simulink model "sgMdl_IO424_SynchroMeasurementTest"  (R2024b)
settings: Solver=FixedStepAuto  StartTime=0.0  StopTime=inf  RelTol=1e-3
libraries: dspsrcs4 x4, speedgoatlib_IO424 x2, speedgoatlib_IO107 x1
Description:
  | IO424 - Synchro Measurement
settings Model: ModifiedByFormat=Speedgoat  Creator=Speedgoat  LastModifiedBy=Speedgoat
settings SolverCC: ConcurrentTasks=on  PositivePriorityOrder=on
settings OptimizationCC: BlockReduction=off  OptimizeBlockIOStorage=off
settings DebuggingCC: TasksWithSamePriorityMsg=none
settings HardwareCC: ProdBitPerLong=64  ProdLongLongMode=on  ProdHWDeviceType=Intel->x86-64 (Linux 64)
settings RTWCC: Description=Speedgoat Real-Time Target Machine  SystemTargetFile=speedgoat.tlc  TemplateMakefile=slrealtime_default_tmf  Toolchain=Simulink Real-Time Toolchain  BuildConfiguration=Faster Runs  TargetLang=C++
settings SimulinkRealTimeTargetCC: SubcomponentCodeInterfacePackaging=Reusable function  InstructionSetFMA=off  LogToMDFFile=off  SLRTFileLogMaxRuns=10
settings ConfigComp: CovBoundaryAbsTol=1.0e-5

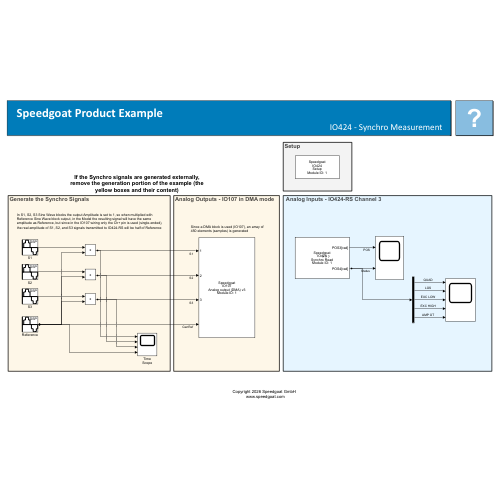
[thumbnail: Simulink's stored preview of the top-level diagram]
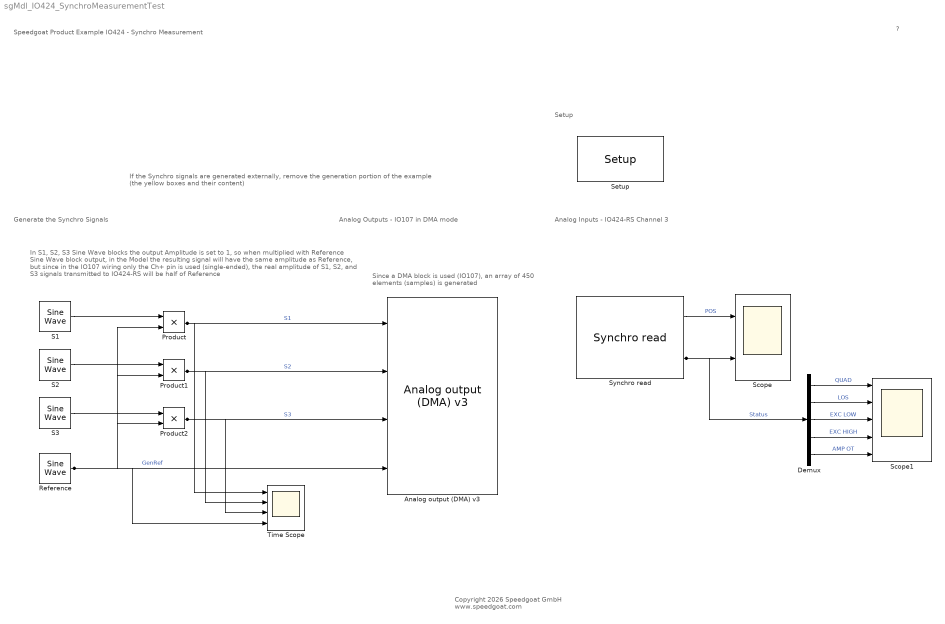
== system sgMdl_IO424_SynchroMeasurementTest ==
  note: Since a DMA block is used (IO107), an array of
      | 450 elements (samples) is generated
  note: If the Synchro signals are generated externally, remove the generation portion of the example (the yellow boxes and their content)
  note: Setup
  note: Generate the Synchro Signals
  note: Analog Inputs - IO424-RS Channel 3
  note: Analog Outputs - IO107 in DMA mode
  note: In S1, S2, S3 Sine Wave blocks the output Amplitude is set to 1, so when multiplied with Reference Sine Wave block output, in the Model the resulting signal will have the same amplitude as Reference, but since in the IO107 wiring only the Ch+ pin is used (single-ended), the real amplitude of S1, S2, and S3 signals transmitted to IO424-RS will be half of Reference
  note: Speedgoat Product Example
      | IO424 - Synchro Measurement
  note: ?
  note: Copyright 2026 Speedgoat GmbH
      |  www.speedgoat.com
  Analog output (DMA) v3 : speedgoatlib_IO107/Analog output (DMA) v3  id=1  slot=-1  channel_str=[1 10 2 11]  range=+-10.0  parInit_str=0  parReset_str=[1]  autocal=on  gsense=off  clksrc=Internal  syncmode=Async (replay function)  extsync=LVDS  framesize_str=450  samplerate_str=450000  sampletime_str=-1
      settings: SourceProductName=IO107
  Demux : Demux  Outputs=5
  Product : Product
  Product1 : Product
  Product2 : Product
  Reference : dspsrcs4/Sine Wave  Amplitude=6.5*sqrt(2)  Frequency=1e3  Phase=0  SampleMode=Discrete  OutComplex=Real  CompMethod=Trigonometric fcn  TableSize=Speed  SampleTime=1/450e3  SamplesPerFrame=450  ResetState=Restart at time zero  OutputFrames=off  dataType=double  wordLen=16  udDataType=sfix(16)  fracBitsMode=Best precision  numFracBits=15  OutDataTypeStr=double  LastOutDataTypeStr=double
  S1 : dspsrcs4/Sine Wave  Amplitude=1  Frequency=10  Phase=pi/2+(2*pi/3)  SampleMode=Discrete  OutComplex=Real  CompMethod=Trigonometric fcn  TableSize=Speed  SampleTime=1/450e3  SamplesPerFrame=450  ResetState=Restart at time zero  OutputFrames=off  dataType=double  wordLen=16  udDataType=sfix(16)  fracBitsMode=Best precision  numFracBits=15  OutDataTypeStr=double  LastOutDataTypeStr=double
  S2 : dspsrcs4/Sine Wave  Amplitude=1  Frequency=10  Phase=pi/2  SampleMode=Discrete  OutComplex=Real  CompMethod=Trigonometric fcn  TableSize=Speed  SampleTime=1/450e3  SamplesPerFrame=450  ResetState=Restart at time zero  OutputFrames=off  dataType=double  wordLen=16  udDataType=sfix(16)  fracBitsMode=Best precision  numFracBits=15  OutDataTypeStr=double  LastOutDataTypeStr=double
  S3 : dspsrcs4/Sine Wave  Amplitude=1  Frequency=10  Phase=pi/2+(4*pi/3)  SampleMode=Discrete  OutComplex=Real  CompMethod=Trigonometric fcn  TableSize=Speed  SampleTime=1/450e3  SamplesPerFrame=450  ResetState=Restart at time zero  OutputFrames=off  dataType=double  wordLen=16  udDataType=sfix(16)  fracBitsMode=Best precision  numFracBits=15  OutDataTypeStr=double  LastOutDataTypeStr=double
  Scope : Scope  NumInputPorts=2
  Scope1 : Scope  NumInputPorts=5
  Setup : speedgoatlib_IO424/Setup  parId=1  parModType=IO424-RS (with Synchro)  parPciSlot=-1  parChConf1=Disabled  parChConf2=Disabled  parChConf3=Synchro  parChConf4=Disabled  parPosRdcUnit=Radiants  parCombRdcCh12=off  parCombRdcCh34=on  parChRdcRange1=3.54 Vrms  parChRdcRange2=7.07 Vrms  parChRdcRange3=14.14 Vrms  parChRdcRange4=14.14 Vrms  parPosSynchroUnit=Radiants  parCombSynchroCh34=on  parChSynchroRange3=14 Vrms  parChSynchroRange4=28 Vrms  parCombLvdtCh12=on  parCombLvdtCh34=on  parLvdtRange1A=7.07 Vrms  parLvdtRange1B=14.14 Vrms  parLvdtRange2A=7.07 Vrms  parLvdtRange2B=14.14 Vrms  parLvdtRange3A=7.07 Vrms  parLvdtRange3B=14.14 Vrms  parLvdtRange4A=7.07 Vrms  parLvdtRange4B=14.14 Vrms  parExcEna1=off  parExcVolt1=2  parExcFreq1=1000  parExcEna2=off  parExcVolt2=2  parExcFreq2=1000  parExcEna3=off  parExcVolt3=2  parExcFreq3=1000  parExcEna4=off  parExcVolt4=2  parExcFreq4=1000
      settings: SourceProductName=IO424
  Synchro read : speedgoatlib_IO424/Synchro read  parId=1  parShowStatus=on  parSampleTime=-1  parOutUnits=1  parChannels=3  parCombCh34=0  parNCh=1
      settings: SourceProductName=IO424
  Time Scope : Scope  NumInputPorts=4
  wires:
  Synchro read/2 -> Demux/1, Scope/2  "Status"
  Synchro read/1 -> Scope/1  "POS"
  Product1/1 -> Time Scope/2, Analog output (DMA) v3/2  "S2"
  Product/1 -> Analog output (DMA) v3/1, Time Scope/1  "S1"
  Reference/1 -> Product2/2, Product1/2, Product/2, Time Scope/4, Analog output (DMA) v3/4  "GenRef"
  S1/1 -> Product/1
  S2/1 -> Product1/1
  Demux/5 -> Scope1/5  "AMP OT"
  Demux/4 -> Scope1/4  "EXC HIGH"
  Demux/1 -> Scope1/1  "QUAD"
  Demux/3 -> Scope1/3  "EXC LOW"
  Demux/2 -> Scope1/2  "LOS"
  S3/1 -> Product2/1
  Product2/1 -> Analog output (DMA) v3/3, Time Scope/3  "S3"
